simulink model "Eigth_Bit_Adder"  (R2023a)
settings: Solver=VariableStepAuto  StartTime=0.0  StopTime=10.0  RelTol=1e-3
settings Model: Creator=MAN  LastModifiedBy=MAN

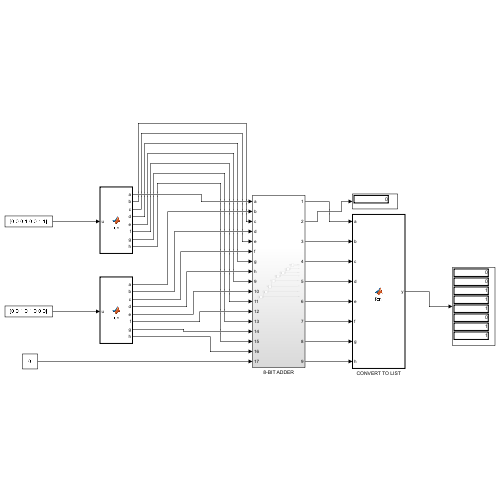
[thumbnail: Simulink's stored preview of the top-level diagram]
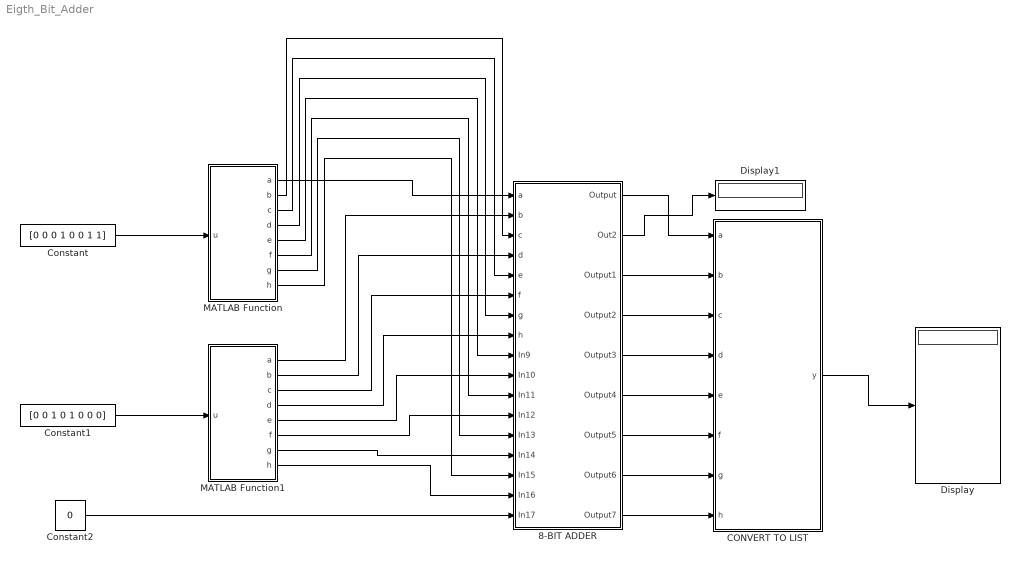
== system Eigth_Bit_Adder ==
  8-BIT ADDER : Subsystem
  CONVERT TO LIST : MATLAB Function  TreatAsAtomicUnit=on
  Constant : Constant  Value=[0 0 0 1 0 0 1 1]
  Constant1 : Constant  Value=[0 0 1 0 1 0 0 0]
  Constant2 : Constant  Value=0
  Display : Display
  Display1 : Display
  MATLAB Function : MATLAB Function  TreatAsAtomicUnit=on
  MATLAB Function1 : MATLAB Function  TreatAsAtomicUnit=on
  wires:
  CONVERT TO LIST/1(y) -> Display/1
  Constant2/1 -> 8-BIT ADDER/17(In17)
  8-BIT ADDER/1(Output) -> CONVERT TO LIST/1(a)
  8-BIT ADDER/3(Output1) -> CONVERT TO LIST/2(b)
  8-BIT ADDER/4(Output2) -> CONVERT TO LIST/3(c)
  8-BIT ADDER/5(Output3) -> CONVERT TO LIST/4(d)
  8-BIT ADDER/6(Output4) -> CONVERT TO LIST/5(e)
  8-BIT ADDER/7(Output5) -> CONVERT TO LIST/6(f)
  8-BIT ADDER/8(Output6) -> CONVERT TO LIST/7(g)
  8-BIT ADDER/9(Output7) -> CONVERT TO LIST/8(h)
  8-BIT ADDER/2(Out2) -> Display1/1
  MATLAB Function/1(a) -> 8-BIT ADDER/1(a)
  MATLAB Function1/1(a) -> 8-BIT ADDER/2(b)
  MATLAB Function/2(b) -> 8-BIT ADDER/3(c)
  MATLAB Function1/2(b) -> 8-BIT ADDER/4(d)
  MATLAB Function/3(c) -> 8-BIT ADDER/5(e)
  MATLAB Function1/3(c) -> 8-BIT ADDER/6(f)
  MATLAB Function/4(d) -> 8-BIT ADDER/7(g)
  MATLAB Function1/4(d) -> 8-BIT ADDER/8(h)
  MATLAB Function/5(e) -> 8-BIT ADDER/9(In9)
  MATLAB Function1/5(e) -> 8-BIT ADDER/10(In10)
  MATLAB Function/6(f) -> 8-BIT ADDER/11(In11)
  MATLAB Function1/6(f) -> 8-BIT ADDER/12(In12)
  MATLAB Function/7(g) -> 8-BIT ADDER/13(In13)
  MATLAB Function1/7(g) -> 8-BIT ADDER/14(In14)
  MATLAB Function/8(h) -> 8-BIT ADDER/15(In15)
  MATLAB Function1/8(h) -> 8-BIT ADDER/16(In16)
  Constant/1 -> MATLAB Function/1(u)
  Constant1/1 -> MATLAB Function1/1(u)

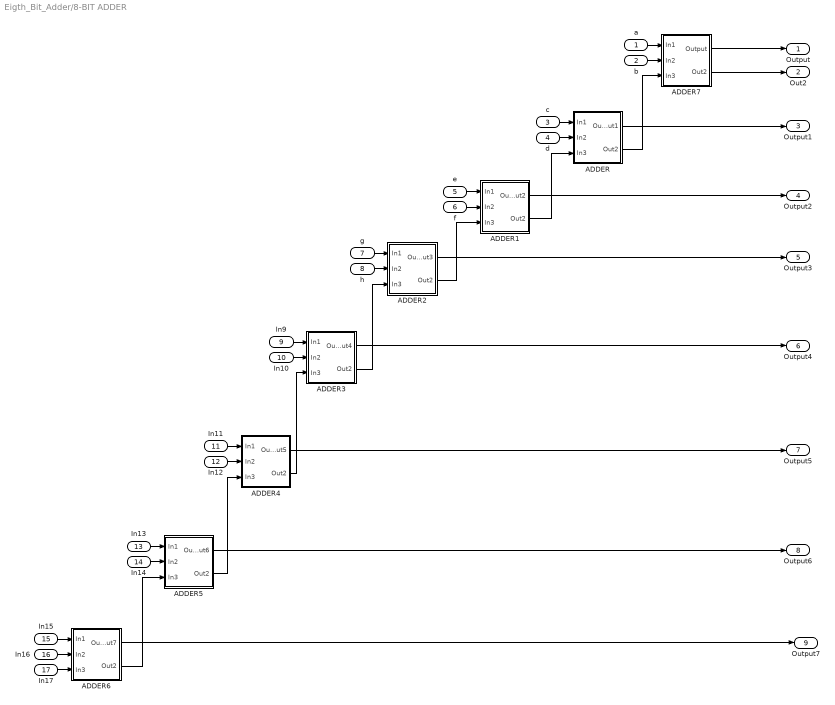
== system Eigth_Bit_Adder/8-BIT ADDER ==
  a : Inport
  b : Inport  Port=2
  c : Inport  Port=3
  d : Inport  Port=4
  e : Inport  Port=5
  f : Inport  Port=6
  g : Inport  Port=7
  h : Inport  Port=8
  In9 : Inport  Port=9
  In10 : Inport  Port=10
  In11 : Inport  Port=11
  In12 : Inport  Port=12
  In13 : Inport  Port=13
  In14 : Inport  Port=14
  In15 : Inport  Port=15
  In16 : Inport  Port=16
  In17 : Inport  Port=17
  ADDER : Subsystem
  ADDER1 : Subsystem
  ADDER2 : Subsystem
  ADDER3 : Subsystem
  ADDER4 : Subsystem
  ADDER5 : Subsystem
  ADDER6 : Subsystem
  ADDER7 : Subsystem
  Output : Outport
  Out2 : Outport  Port=2
  Output1 : Outport  Port=3
  Output2 : Outport  Port=4
  Output3 : Outport  Port=5
  Output4 : Outport  Port=6
  Output5 : Outport  Port=7
  Output6 : Outport  Port=8
  Output7 : Outport  Port=9
  wires:
  ADDER3/1(Output4) -> Output4/1
  ADDER1/2(Out2) -> ADDER/3(In3)
  h/1 -> ADDER2/2(In2)
  In17/1 -> ADDER6/3(In3)
  ADDER/1(Output1) -> Output1/1
  ADDER2/2(Out2) -> ADDER1/3(In3)
  ADDER6/2(Out2) -> ADDER5/3(In3)
  ADDER3/2(Out2) -> ADDER2/3(In3)
  In16/1 -> ADDER6/2(In2)
  ADDER4/2(Out2) -> ADDER3/3(In3)
  In10/1 -> ADDER3/2(In2)
  ADDER5/2(Out2) -> ADDER4/3(In3)
  ADDER2/1(Output3) -> Output3/1
  In14/1 -> ADDER5/2(In2)
  ADDER6/1(Output7) -> Output7/1
  ADDER/2(Out2) -> ADDER7/3(In3)
  ADDER5/1(Output6) -> Output6/1
  ADDER1/1(Output2) -> Output2/1
  f/1 -> ADDER1/2(In2)
  In9/1 -> ADDER3/1(In1)
  e/1 -> ADDER1/1(In1)
  c/1 -> ADDER/1(In1)
  ADDER7/1(Output) -> Output/1
  g/1 -> ADDER2/1(In1)
  d/1 -> ADDER/2(In2)
  a/1 -> ADDER7/1(In1)
  b/1 -> ADDER7/2(In2)
  In12/1 -> ADDER4/2(In2)
  ADDER7/2(Out2) -> Out2/1
  In15/1 -> ADDER6/1(In1)
  In11/1 -> ADDER4/1(In1)
  In13/1 -> ADDER5/1(In1)
  ADDER4/1(Output5) -> Output5/1

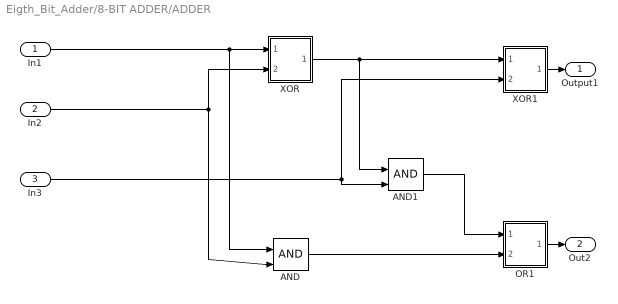
== system Eigth_Bit_Adder/8-BIT ADDER/ADDER ==
  In1 : Inport
  In2 : Inport  Port=2
  In3 : Inport  Port=3
  AND : Logic  IconShape=distinctive  AllPortsSameDT=off  OutDataTypeStr=boolean
  AND1 : Logic  IconShape=distinctive  AllPortsSameDT=off  OutDataTypeStr=boolean
  OR1 : Subsystem
  XOR : Subsystem
  XOR1 : Subsystem
  Output1 : Outport
  Out2 : Outport  Port=2
  wires:
  XOR/1(Out1) -> AND1/1, XOR1/1(In1)
  AND/1 -> OR1/2(In2)
  In2/1 -> XOR/2(In2), AND/2
  In3/1 -> XOR1/2(In2), AND1/2
  In1/1 -> AND/1, XOR/1(In1)
  OR1/1(Out1) -> Out2/1
  AND1/1 -> OR1/1(In1)
  XOR1/1(Out1) -> Output1/1

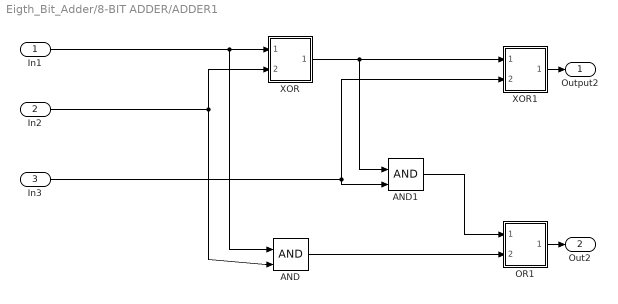
== system Eigth_Bit_Adder/8-BIT ADDER/ADDER1 ==
  In1 : Inport
  In2 : Inport  Port=2
  In3 : Inport  Port=3
  AND : Logic  IconShape=distinctive  AllPortsSameDT=off  OutDataTypeStr=boolean
  AND1 : Logic  IconShape=distinctive  AllPortsSameDT=off  OutDataTypeStr=boolean
  OR1 : Subsystem
  XOR : Subsystem
  XOR1 : Subsystem
  Output2 : Outport
  Out2 : Outport  Port=2
  wires:
  XOR/1(Out1) -> AND1/1, XOR1/1(In1)
  AND/1 -> OR1/2(In2)
  In2/1 -> XOR/2(In2), AND/2
  In3/1 -> XOR1/2(In2), AND1/2
  In1/1 -> AND/1, XOR/1(In1)
  OR1/1(Out1) -> Out2/1
  AND1/1 -> OR1/1(In1)
  XOR1/1(Out1) -> Output2/1

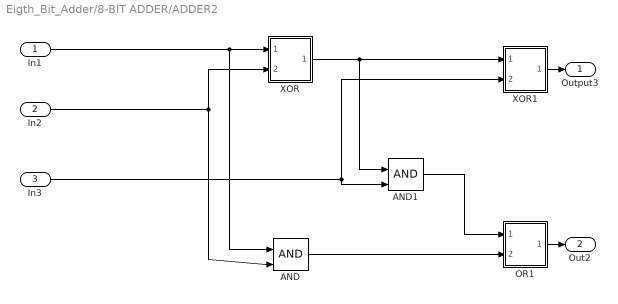
== system Eigth_Bit_Adder/8-BIT ADDER/ADDER2 ==
  In1 : Inport
  In2 : Inport  Port=2
  In3 : Inport  Port=3
  AND : Logic  IconShape=distinctive  AllPortsSameDT=off  OutDataTypeStr=boolean
  AND1 : Logic  IconShape=distinctive  AllPortsSameDT=off  OutDataTypeStr=boolean
  OR1 : Subsystem
  XOR : Subsystem
  XOR1 : Subsystem
  Output3 : Outport
  Out2 : Outport  Port=2
  wires:
  XOR/1(Out1) -> AND1/1, XOR1/1(In1)
  AND/1 -> OR1/2(In2)
  In2/1 -> XOR/2(In2), AND/2
  In3/1 -> XOR1/2(In2), AND1/2
  In1/1 -> AND/1, XOR/1(In1)
  OR1/1(Out1) -> Out2/1
  AND1/1 -> OR1/1(In1)
  XOR1/1(Out1) -> Output3/1

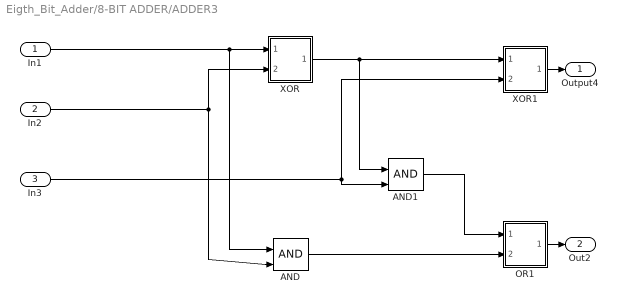
== system Eigth_Bit_Adder/8-BIT ADDER/ADDER3 ==
  In1 : Inport
  In2 : Inport  Port=2
  In3 : Inport  Port=3
  AND : Logic  IconShape=distinctive  AllPortsSameDT=off  OutDataTypeStr=boolean
  AND1 : Logic  IconShape=distinctive  AllPortsSameDT=off  OutDataTypeStr=boolean
  OR1 : Subsystem
  XOR : Subsystem
  XOR1 : Subsystem
  Output4 : Outport
  Out2 : Outport  Port=2
  wires:
  XOR/1(Out1) -> AND1/1, XOR1/1(In1)
  AND/1 -> OR1/2(In2)
  In2/1 -> XOR/2(In2), AND/2
  In3/1 -> XOR1/2(In2), AND1/2
  In1/1 -> AND/1, XOR/1(In1)
  OR1/1(Out1) -> Out2/1
  AND1/1 -> OR1/1(In1)
  XOR1/1(Out1) -> Output4/1

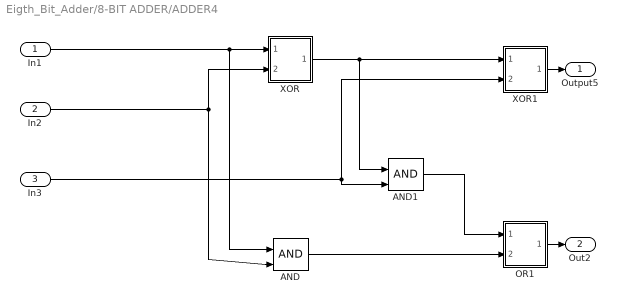
== system Eigth_Bit_Adder/8-BIT ADDER/ADDER4 ==
  In1 : Inport
  In2 : Inport  Port=2
  In3 : Inport  Port=3
  AND : Logic  IconShape=distinctive  AllPortsSameDT=off  OutDataTypeStr=boolean
  AND1 : Logic  IconShape=distinctive  AllPortsSameDT=off  OutDataTypeStr=boolean
  OR1 : Subsystem
  XOR : Subsystem
  XOR1 : Subsystem
  Output5 : Outport
  Out2 : Outport  Port=2
  wires:
  XOR/1(Out1) -> AND1/1, XOR1/1(In1)
  AND/1 -> OR1/2(In2)
  In2/1 -> XOR/2(In2), AND/2
  In3/1 -> XOR1/2(In2), AND1/2
  In1/1 -> AND/1, XOR/1(In1)
  OR1/1(Out1) -> Out2/1
  AND1/1 -> OR1/1(In1)
  XOR1/1(Out1) -> Output5/1

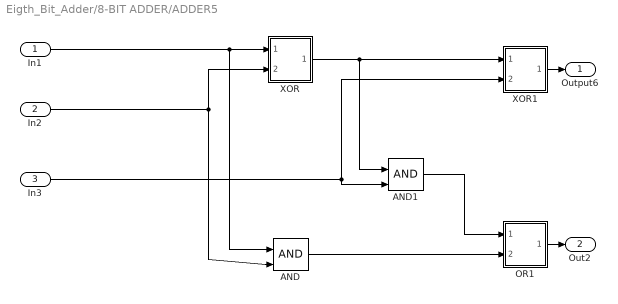
== system Eigth_Bit_Adder/8-BIT ADDER/ADDER5 ==
  In1 : Inport
  In2 : Inport  Port=2
  In3 : Inport  Port=3
  AND : Logic  IconShape=distinctive  AllPortsSameDT=off  OutDataTypeStr=boolean
  AND1 : Logic  IconShape=distinctive  AllPortsSameDT=off  OutDataTypeStr=boolean
  OR1 : Subsystem
  XOR : Subsystem
  XOR1 : Subsystem
  Output6 : Outport
  Out2 : Outport  Port=2
  wires:
  XOR/1(Out1) -> AND1/1, XOR1/1(In1)
  AND/1 -> OR1/2(In2)
  In2/1 -> XOR/2(In2), AND/2
  In3/1 -> XOR1/2(In2), AND1/2
  In1/1 -> AND/1, XOR/1(In1)
  OR1/1(Out1) -> Out2/1
  AND1/1 -> OR1/1(In1)
  XOR1/1(Out1) -> Output6/1

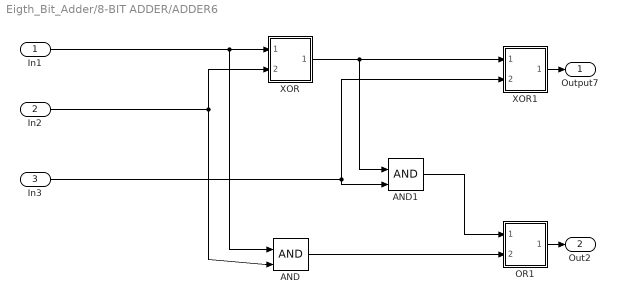
== system Eigth_Bit_Adder/8-BIT ADDER/ADDER6 ==
  In1 : Inport
  In2 : Inport  Port=2
  In3 : Inport  Port=3
  AND : Logic  IconShape=distinctive  AllPortsSameDT=off  OutDataTypeStr=boolean
  AND1 : Logic  IconShape=distinctive  AllPortsSameDT=off  OutDataTypeStr=boolean
  OR1 : Subsystem
  XOR : Subsystem
  XOR1 : Subsystem
  Output7 : Outport
  Out2 : Outport  Port=2
  wires:
  XOR/1(Out1) -> AND1/1, XOR1/1(In1)
  AND/1 -> OR1/2(In2)
  In2/1 -> XOR/2(In2), AND/2
  In3/1 -> XOR1/2(In2), AND1/2
  In1/1 -> AND/1, XOR/1(In1)
  OR1/1(Out1) -> Out2/1
  AND1/1 -> OR1/1(In1)
  XOR1/1(Out1) -> Output7/1

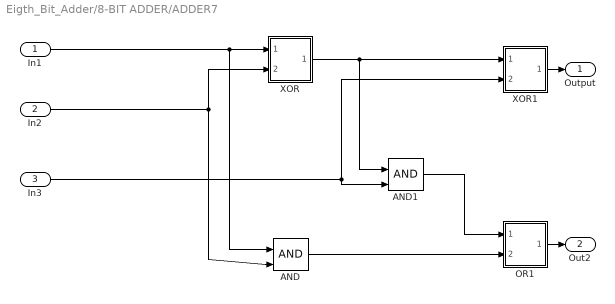
== system Eigth_Bit_Adder/8-BIT ADDER/ADDER7 ==
  In1 : Inport
  In2 : Inport  Port=2
  In3 : Inport  Port=3
  AND : Logic  IconShape=distinctive  AllPortsSameDT=off  OutDataTypeStr=boolean
  AND1 : Logic  IconShape=distinctive  AllPortsSameDT=off  OutDataTypeStr=boolean
  OR1 : Subsystem
  XOR : Subsystem
  XOR1 : Subsystem
  Output : Outport
  Out2 : Outport  Port=2
  wires:
  XOR/1(Out1) -> AND1/1, XOR1/1(In1)
  AND/1 -> OR1/2(In2)
  In2/1 -> XOR/2(In2), AND/2
  In3/1 -> XOR1/2(In2), AND1/2
  In1/1 -> AND/1, XOR/1(In1)
  OR1/1(Out1) -> Out2/1
  AND1/1 -> OR1/1(In1)
  XOR1/1(Out1) -> Output/1

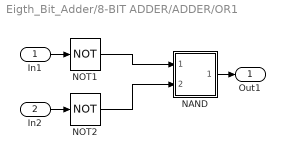
== system Eigth_Bit_Adder/8-BIT ADDER/ADDER/OR1 ==
  In1 : Inport
  In2 : Inport  Port=2
  NAND : Subsystem
  NOT1 : Logic  Operator=NOT  IconShape=distinctive  AllPortsSameDT=off  OutDataTypeStr=boolean
  NOT2 : Logic  Operator=NOT  IconShape=distinctive  AllPortsSameDT=off  OutDataTypeStr=boolean
  Out1 : Outport
  wires:
  In1/1 -> NOT1/1
  In2/1 -> NOT2/1
  NOT1/1 -> NAND/1(In1)
  NOT2/1 -> NAND/2(In2)
  NAND/1(Out1) -> Out1/1

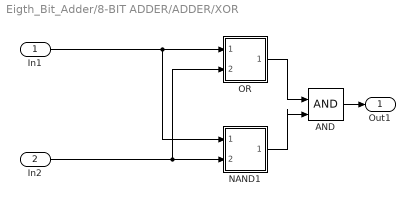
== system Eigth_Bit_Adder/8-BIT ADDER/ADDER/XOR ==
  In1 : Inport
  In2 : Inport  Port=2
  AND : Logic  IconShape=distinctive  AllPortsSameDT=off  OutDataTypeStr=boolean
  NAND1 : Subsystem
  OR : Subsystem
  Out1 : Outport
  wires:
  In2/1 -> NAND1/2(In2), OR/2(In2)
  In1/1 -> NAND1/1(In1), OR/1(In1)
  NAND1/1(Out1) -> AND/2
  AND/1 -> Out1/1
  OR/1(Out1) -> AND/1

== system Eigth_Bit_Adder/8-BIT ADDER/ADDER/XOR1 ==
  In1 : Inport
  In2 : Inport  Port=2
  AND : Logic  IconShape=distinctive  AllPortsSameDT=off  OutDataTypeStr=boolean
  NAND1 : Subsystem
  OR : Subsystem
  Out1 : Outport
  wires:
  In2/1 -> NAND1/2(In2), OR/2(In2)
  In1/1 -> NAND1/1(In1), OR/1(In1)
  NAND1/1(Out1) -> AND/2
  AND/1 -> Out1/1
  OR/1(Out1) -> AND/1

== system Eigth_Bit_Adder/8-BIT ADDER/ADDER1/OR1 ==
  In1 : Inport
  In2 : Inport  Port=2
  NAND : Subsystem
  NOT1 : Logic  Operator=NOT  IconShape=distinctive  AllPortsSameDT=off  OutDataTypeStr=boolean
  NOT2 : Logic  Operator=NOT  IconShape=distinctive  AllPortsSameDT=off  OutDataTypeStr=boolean
  Out1 : Outport
  wires:
  In1/1 -> NOT1/1
  In2/1 -> NOT2/1
  NOT1/1 -> NAND/1(In1)
  NOT2/1 -> NAND/2(In2)
  NAND/1(Out1) -> Out1/1

== system Eigth_Bit_Adder/8-BIT ADDER/ADDER1/XOR ==
  In1 : Inport
  In2 : Inport  Port=2
  AND : Logic  IconShape=distinctive  AllPortsSameDT=off  OutDataTypeStr=boolean
  NAND1 : Subsystem
  OR : Subsystem
  Out1 : Outport
  wires:
  In2/1 -> NAND1/2(In2), OR/2(In2)
  In1/1 -> NAND1/1(In1), OR/1(In1)
  NAND1/1(Out1) -> AND/2
  AND/1 -> Out1/1
  OR/1(Out1) -> AND/1

== system Eigth_Bit_Adder/8-BIT ADDER/ADDER1/XOR1 ==
  In1 : Inport
  In2 : Inport  Port=2
  AND : Logic  IconShape=distinctive  AllPortsSameDT=off  OutDataTypeStr=boolean
  NAND1 : Subsystem
  OR : Subsystem
  Out1 : Outport
  wires:
  In2/1 -> NAND1/2(In2), OR/2(In2)
  In1/1 -> NAND1/1(In1), OR/1(In1)
  NAND1/1(Out1) -> AND/2
  AND/1 -> Out1/1
  OR/1(Out1) -> AND/1

== system Eigth_Bit_Adder/8-BIT ADDER/ADDER2/OR1 ==
  In1 : Inport
  In2 : Inport  Port=2
  NAND : Subsystem
  NOT1 : Logic  Operator=NOT  IconShape=distinctive  AllPortsSameDT=off  OutDataTypeStr=boolean
  NOT2 : Logic  Operator=NOT  IconShape=distinctive  AllPortsSameDT=off  OutDataTypeStr=boolean
  Out1 : Outport
  wires:
  In1/1 -> NOT1/1
  In2/1 -> NOT2/1
  NOT1/1 -> NAND/1(In1)
  NOT2/1 -> NAND/2(In2)
  NAND/1(Out1) -> Out1/1

== system Eigth_Bit_Adder/8-BIT ADDER/ADDER2/XOR ==
  In1 : Inport
  In2 : Inport  Port=2
  AND : Logic  IconShape=distinctive  AllPortsSameDT=off  OutDataTypeStr=boolean
  NAND1 : Subsystem
  OR : Subsystem
  Out1 : Outport
  wires:
  In2/1 -> NAND1/2(In2), OR/2(In2)
  In1/1 -> NAND1/1(In1), OR/1(In1)
  NAND1/1(Out1) -> AND/2
  AND/1 -> Out1/1
  OR/1(Out1) -> AND/1

== system Eigth_Bit_Adder/8-BIT ADDER/ADDER2/XOR1 ==
  In1 : Inport
  In2 : Inport  Port=2
  AND : Logic  IconShape=distinctive  AllPortsSameDT=off  OutDataTypeStr=boolean
  NAND1 : Subsystem
  OR : Subsystem
  Out1 : Outport
  wires:
  In2/1 -> NAND1/2(In2), OR/2(In2)
  In1/1 -> NAND1/1(In1), OR/1(In1)
  NAND1/1(Out1) -> AND/2
  AND/1 -> Out1/1
  OR/1(Out1) -> AND/1

== system Eigth_Bit_Adder/8-BIT ADDER/ADDER3/OR1 ==
  In1 : Inport
  In2 : Inport  Port=2
  NAND : Subsystem
  NOT1 : Logic  Operator=NOT  IconShape=distinctive  AllPortsSameDT=off  OutDataTypeStr=boolean
  NOT2 : Logic  Operator=NOT  IconShape=distinctive  AllPortsSameDT=off  OutDataTypeStr=boolean
  Out1 : Outport
  wires:
  In1/1 -> NOT1/1
  In2/1 -> NOT2/1
  NOT1/1 -> NAND/1(In1)
  NOT2/1 -> NAND/2(In2)
  NAND/1(Out1) -> Out1/1

== system Eigth_Bit_Adder/8-BIT ADDER/ADDER3/XOR ==
  In1 : Inport
  In2 : Inport  Port=2
  AND : Logic  IconShape=distinctive  AllPortsSameDT=off  OutDataTypeStr=boolean
  NAND1 : Subsystem
  OR : Subsystem
  Out1 : Outport
  wires:
  In2/1 -> NAND1/2(In2), OR/2(In2)
  In1/1 -> NAND1/1(In1), OR/1(In1)
  NAND1/1(Out1) -> AND/2
  AND/1 -> Out1/1
  OR/1(Out1) -> AND/1

== system Eigth_Bit_Adder/8-BIT ADDER/ADDER3/XOR1 ==
  In1 : Inport
  In2 : Inport  Port=2
  AND : Logic  IconShape=distinctive  AllPortsSameDT=off  OutDataTypeStr=boolean
  NAND1 : Subsystem
  OR : Subsystem
  Out1 : Outport
  wires:
  In2/1 -> NAND1/2(In2), OR/2(In2)
  In1/1 -> NAND1/1(In1), OR/1(In1)
  NAND1/1(Out1) -> AND/2
  AND/1 -> Out1/1
  OR/1(Out1) -> AND/1

== system Eigth_Bit_Adder/8-BIT ADDER/ADDER4/OR1 ==
  In1 : Inport
  In2 : Inport  Port=2
  NAND : Subsystem
  NOT1 : Logic  Operator=NOT  IconShape=distinctive  AllPortsSameDT=off  OutDataTypeStr=boolean
  NOT2 : Logic  Operator=NOT  IconShape=distinctive  AllPortsSameDT=off  OutDataTypeStr=boolean
  Out1 : Outport
  wires:
  In1/1 -> NOT1/1
  In2/1 -> NOT2/1
  NOT1/1 -> NAND/1(In1)
  NOT2/1 -> NAND/2(In2)
  NAND/1(Out1) -> Out1/1

== system Eigth_Bit_Adder/8-BIT ADDER/ADDER4/XOR ==
  In1 : Inport
  In2 : Inport  Port=2
  AND : Logic  IconShape=distinctive  AllPortsSameDT=off  OutDataTypeStr=boolean
  NAND1 : Subsystem
  OR : Subsystem
  Out1 : Outport
  wires:
  In2/1 -> NAND1/2(In2), OR/2(In2)
  In1/1 -> NAND1/1(In1), OR/1(In1)
  NAND1/1(Out1) -> AND/2
  AND/1 -> Out1/1
  OR/1(Out1) -> AND/1

== system Eigth_Bit_Adder/8-BIT ADDER/ADDER4/XOR1 ==
  In1 : Inport
  In2 : Inport  Port=2
  AND : Logic  IconShape=distinctive  AllPortsSameDT=off  OutDataTypeStr=boolean
  NAND1 : Subsystem
  OR : Subsystem
  Out1 : Outport
  wires:
  In2/1 -> NAND1/2(In2), OR/2(In2)
  In1/1 -> NAND1/1(In1), OR/1(In1)
  NAND1/1(Out1) -> AND/2
  AND/1 -> Out1/1
  OR/1(Out1) -> AND/1

== system Eigth_Bit_Adder/8-BIT ADDER/ADDER5/OR1 ==
  In1 : Inport
  In2 : Inport  Port=2
  NAND : Subsystem
  NOT1 : Logic  Operator=NOT  IconShape=distinctive  AllPortsSameDT=off  OutDataTypeStr=boolean
  NOT2 : Logic  Operator=NOT  IconShape=distinctive  AllPortsSameDT=off  OutDataTypeStr=boolean
  Out1 : Outport
  wires:
  In1/1 -> NOT1/1
  In2/1 -> NOT2/1
  NOT1/1 -> NAND/1(In1)
  NOT2/1 -> NAND/2(In2)
  NAND/1(Out1) -> Out1/1

== system Eigth_Bit_Adder/8-BIT ADDER/ADDER5/XOR ==
  In1 : Inport
  In2 : Inport  Port=2
  AND : Logic  IconShape=distinctive  AllPortsSameDT=off  OutDataTypeStr=boolean
  NAND1 : Subsystem
  OR : Subsystem
  Out1 : Outport
  wires:
  In2/1 -> NAND1/2(In2), OR/2(In2)
  In1/1 -> NAND1/1(In1), OR/1(In1)
  NAND1/1(Out1) -> AND/2
  AND/1 -> Out1/1
  OR/1(Out1) -> AND/1

== system Eigth_Bit_Adder/8-BIT ADDER/ADDER5/XOR1 ==
  In1 : Inport
  In2 : Inport  Port=2
  AND : Logic  IconShape=distinctive  AllPortsSameDT=off  OutDataTypeStr=boolean
  NAND1 : Subsystem
  OR : Subsystem
  Out1 : Outport
  wires:
  In2/1 -> NAND1/2(In2), OR/2(In2)
  In1/1 -> NAND1/1(In1), OR/1(In1)
  NAND1/1(Out1) -> AND/2
  AND/1 -> Out1/1
  OR/1(Out1) -> AND/1

== system Eigth_Bit_Adder/8-BIT ADDER/ADDER6/OR1 ==
  In1 : Inport
  In2 : Inport  Port=2
  NAND : Subsystem
  NOT1 : Logic  Operator=NOT  IconShape=distinctive  AllPortsSameDT=off  OutDataTypeStr=boolean
  NOT2 : Logic  Operator=NOT  IconShape=distinctive  AllPortsSameDT=off  OutDataTypeStr=boolean
  Out1 : Outport
  wires:
  In1/1 -> NOT1/1
  In2/1 -> NOT2/1
  NOT1/1 -> NAND/1(In1)
  NOT2/1 -> NAND/2(In2)
  NAND/1(Out1) -> Out1/1

== system Eigth_Bit_Adder/8-BIT ADDER/ADDER6/XOR ==
  In1 : Inport
  In2 : Inport  Port=2
  AND : Logic  IconShape=distinctive  AllPortsSameDT=off  OutDataTypeStr=boolean
  NAND1 : Subsystem
  OR : Subsystem
  Out1 : Outport
  wires:
  In2/1 -> NAND1/2(In2), OR/2(In2)
  In1/1 -> NAND1/1(In1), OR/1(In1)
  NAND1/1(Out1) -> AND/2
  AND/1 -> Out1/1
  OR/1(Out1) -> AND/1

== system Eigth_Bit_Adder/8-BIT ADDER/ADDER6/XOR1 ==
  In1 : Inport
  In2 : Inport  Port=2
  AND : Logic  IconShape=distinctive  AllPortsSameDT=off  OutDataTypeStr=boolean
  NAND1 : Subsystem
  OR : Subsystem
  Out1 : Outport
  wires:
  In2/1 -> NAND1/2(In2), OR/2(In2)
  In1/1 -> NAND1/1(In1), OR/1(In1)
  NAND1/1(Out1) -> AND/2
  AND/1 -> Out1/1
  OR/1(Out1) -> AND/1

== system Eigth_Bit_Adder/8-BIT ADDER/ADDER7/OR1 ==
  In1 : Inport
  In2 : Inport  Port=2
  NAND : Subsystem
  NOT1 : Logic  Operator=NOT  IconShape=distinctive  AllPortsSameDT=off  OutDataTypeStr=boolean
  NOT2 : Logic  Operator=NOT  IconShape=distinctive  AllPortsSameDT=off  OutDataTypeStr=boolean
  Out1 : Outport
  wires:
  In1/1 -> NOT1/1
  In2/1 -> NOT2/1
  NOT1/1 -> NAND/1(In1)
  NOT2/1 -> NAND/2(In2)
  NAND/1(Out1) -> Out1/1

== system Eigth_Bit_Adder/8-BIT ADDER/ADDER7/XOR ==
  In1 : Inport
  In2 : Inport  Port=2
  AND : Logic  IconShape=distinctive  AllPortsSameDT=off  OutDataTypeStr=boolean
  NAND1 : Subsystem
  OR : Subsystem
  Out1 : Outport
  wires:
  In2/1 -> NAND1/2(In2), OR/2(In2)
  In1/1 -> NAND1/1(In1), OR/1(In1)
  NAND1/1(Out1) -> AND/2
  AND/1 -> Out1/1
  OR/1(Out1) -> AND/1

== system Eigth_Bit_Adder/8-BIT ADDER/ADDER7/XOR1 ==
  In1 : Inport
  In2 : Inport  Port=2
  AND : Logic  IconShape=distinctive  AllPortsSameDT=off  OutDataTypeStr=boolean
  NAND1 : Subsystem
  OR : Subsystem
  Out1 : Outport
  wires:
  In2/1 -> NAND1/2(In2), OR/2(In2)
  In1/1 -> NAND1/1(In1), OR/1(In1)
  NAND1/1(Out1) -> AND/2
  AND/1 -> Out1/1
  OR/1(Out1) -> AND/1

== system Eigth_Bit_Adder/8-BIT ADDER/ADDER/OR1/NAND ==
  In1 : Inport
  In2 : Inport  Port=2
  AND : Logic  IconShape=distinctive  AllPortsSameDT=off  OutDataTypeStr=boolean
  NOT : Logic  Operator=NOT  IconShape=distinctive  AllPortsSameDT=off  OutDataTypeStr=boolean
  Out1 : Outport
  wires:
  AND/1 -> NOT/1
  In1/1 -> AND/1
  NOT/1 -> Out1/1
  In2/1 -> AND/2

== system Eigth_Bit_Adder/8-BIT ADDER/ADDER/XOR/NAND1 ==
  In1 : Inport
  In2 : Inport  Port=2
  AND : Logic  IconShape=distinctive  AllPortsSameDT=off  OutDataTypeStr=boolean
  NOT : Logic  Operator=NOT  IconShape=distinctive  AllPortsSameDT=off  OutDataTypeStr=boolean
  Out1 : Outport
  wires:
  In2/1 -> AND/2
  NOT/1 -> Out1/1
  In1/1 -> AND/1
  AND/1 -> NOT/1

== system Eigth_Bit_Adder/8-BIT ADDER/ADDER/XOR/OR ==
  In1 : Inport
  In2 : Inport  Port=2
  NAND : Subsystem
  NOT1 : Logic  Operator=NOT  IconShape=distinctive  AllPortsSameDT=off  OutDataTypeStr=boolean
  NOT2 : Logic  Operator=NOT  IconShape=distinctive  AllPortsSameDT=off  OutDataTypeStr=boolean
  Out1 : Outport
  wires:
  In1/1 -> NOT1/1
  In2/1 -> NOT2/1
  NOT1/1 -> NAND/1(In1)
  NOT2/1 -> NAND/2(In2)
  NAND/1(Out1) -> Out1/1

== system Eigth_Bit_Adder/8-BIT ADDER/ADDER/XOR1/NAND1 ==
  In1 : Inport
  In2 : Inport  Port=2
  AND : Logic  IconShape=distinctive  AllPortsSameDT=off  OutDataTypeStr=boolean
  NOT : Logic  Operator=NOT  IconShape=distinctive  AllPortsSameDT=off  OutDataTypeStr=boolean
  Out1 : Outport
  wires:
  In2/1 -> AND/2
  NOT/1 -> Out1/1
  In1/1 -> AND/1
  AND/1 -> NOT/1

== system Eigth_Bit_Adder/8-BIT ADDER/ADDER/XOR1/OR ==
  In1 : Inport
  In2 : Inport  Port=2
  NAND : Subsystem
  NOT1 : Logic  Operator=NOT  IconShape=distinctive  AllPortsSameDT=off  OutDataTypeStr=boolean
  NOT2 : Logic  Operator=NOT  IconShape=distinctive  AllPortsSameDT=off  OutDataTypeStr=boolean
  Out1 : Outport
  wires:
  In1/1 -> NOT1/1
  In2/1 -> NOT2/1
  NOT1/1 -> NAND/1(In1)
  NOT2/1 -> NAND/2(In2)
  NAND/1(Out1) -> Out1/1

== system Eigth_Bit_Adder/8-BIT ADDER/ADDER1/OR1/NAND ==
  In1 : Inport
  In2 : Inport  Port=2
  AND : Logic  IconShape=distinctive  AllPortsSameDT=off  OutDataTypeStr=boolean
  NOT : Logic  Operator=NOT  IconShape=distinctive  AllPortsSameDT=off  OutDataTypeStr=boolean
  Out1 : Outport
  wires:
  AND/1 -> NOT/1
  In1/1 -> AND/1
  NOT/1 -> Out1/1
  In2/1 -> AND/2

== system Eigth_Bit_Adder/8-BIT ADDER/ADDER1/XOR/NAND1 ==
  In1 : Inport
  In2 : Inport  Port=2
  AND : Logic  IconShape=distinctive  AllPortsSameDT=off  OutDataTypeStr=boolean
  NOT : Logic  Operator=NOT  IconShape=distinctive  AllPortsSameDT=off  OutDataTypeStr=boolean
  Out1 : Outport
  wires:
  In2/1 -> AND/2
  NOT/1 -> Out1/1
  In1/1 -> AND/1
  AND/1 -> NOT/1

== system Eigth_Bit_Adder/8-BIT ADDER/ADDER1/XOR/OR ==
  In1 : Inport
  In2 : Inport  Port=2
  NAND : Subsystem
  NOT1 : Logic  Operator=NOT  IconShape=distinctive  AllPortsSameDT=off  OutDataTypeStr=boolean
  NOT2 : Logic  Operator=NOT  IconShape=distinctive  AllPortsSameDT=off  OutDataTypeStr=boolean
  Out1 : Outport
  wires:
  In1/1 -> NOT1/1
  In2/1 -> NOT2/1
  NOT1/1 -> NAND/1(In1)
  NOT2/1 -> NAND/2(In2)
  NAND/1(Out1) -> Out1/1

== system Eigth_Bit_Adder/8-BIT ADDER/ADDER1/XOR1/NAND1 ==
  In1 : Inport
  In2 : Inport  Port=2
  AND : Logic  IconShape=distinctive  AllPortsSameDT=off  OutDataTypeStr=boolean
  NOT : Logic  Operator=NOT  IconShape=distinctive  AllPortsSameDT=off  OutDataTypeStr=boolean
  Out1 : Outport
  wires:
  In2/1 -> AND/2
  NOT/1 -> Out1/1
  In1/1 -> AND/1
  AND/1 -> NOT/1

== system Eigth_Bit_Adder/8-BIT ADDER/ADDER1/XOR1/OR ==
  In1 : Inport
  In2 : Inport  Port=2
  NAND : Subsystem
  NOT1 : Logic  Operator=NOT  IconShape=distinctive  AllPortsSameDT=off  OutDataTypeStr=boolean
  NOT2 : Logic  Operator=NOT  IconShape=distinctive  AllPortsSameDT=off  OutDataTypeStr=boolean
  Out1 : Outport
  wires:
  In1/1 -> NOT1/1
  In2/1 -> NOT2/1
  NOT1/1 -> NAND/1(In1)
  NOT2/1 -> NAND/2(In2)
  NAND/1(Out1) -> Out1/1

== system Eigth_Bit_Adder/8-BIT ADDER/ADDER2/OR1/NAND ==
  In1 : Inport
  In2 : Inport  Port=2
  AND : Logic  IconShape=distinctive  AllPortsSameDT=off  OutDataTypeStr=boolean
  NOT : Logic  Operator=NOT  IconShape=distinctive  AllPortsSameDT=off  OutDataTypeStr=boolean
  Out1 : Outport
  wires:
  AND/1 -> NOT/1
  In1/1 -> AND/1
  NOT/1 -> Out1/1
  In2/1 -> AND/2

== system Eigth_Bit_Adder/8-BIT ADDER/ADDER2/XOR/NAND1 ==
  In1 : Inport
  In2 : Inport  Port=2
  AND : Logic  IconShape=distinctive  AllPortsSameDT=off  OutDataTypeStr=boolean
  NOT : Logic  Operator=NOT  IconShape=distinctive  AllPortsSameDT=off  OutDataTypeStr=boolean
  Out1 : Outport
  wires:
  In2/1 -> AND/2
  NOT/1 -> Out1/1
  In1/1 -> AND/1
  AND/1 -> NOT/1

== system Eigth_Bit_Adder/8-BIT ADDER/ADDER2/XOR/OR ==
  In1 : Inport
  In2 : Inport  Port=2
  NAND : Subsystem
  NOT1 : Logic  Operator=NOT  IconShape=distinctive  AllPortsSameDT=off  OutDataTypeStr=boolean
  NOT2 : Logic  Operator=NOT  IconShape=distinctive  AllPortsSameDT=off  OutDataTypeStr=boolean
  Out1 : Outport
  wires:
  In1/1 -> NOT1/1
  In2/1 -> NOT2/1
  NOT1/1 -> NAND/1(In1)
  NOT2/1 -> NAND/2(In2)
  NAND/1(Out1) -> Out1/1

== system Eigth_Bit_Adder/8-BIT ADDER/ADDER2/XOR1/NAND1 ==
  In1 : Inport
  In2 : Inport  Port=2
  AND : Logic  IconShape=distinctive  AllPortsSameDT=off  OutDataTypeStr=boolean
  NOT : Logic  Operator=NOT  IconShape=distinctive  AllPortsSameDT=off  OutDataTypeStr=boolean
  Out1 : Outport
  wires:
  In2/1 -> AND/2
  NOT/1 -> Out1/1
  In1/1 -> AND/1
  AND/1 -> NOT/1

== system Eigth_Bit_Adder/8-BIT ADDER/ADDER2/XOR1/OR ==
  In1 : Inport
  In2 : Inport  Port=2
  NAND : Subsystem
  NOT1 : Logic  Operator=NOT  IconShape=distinctive  AllPortsSameDT=off  OutDataTypeStr=boolean
  NOT2 : Logic  Operator=NOT  IconShape=distinctive  AllPortsSameDT=off  OutDataTypeStr=boolean
  Out1 : Outport
  wires:
  In1/1 -> NOT1/1
  In2/1 -> NOT2/1
  NOT1/1 -> NAND/1(In1)
  NOT2/1 -> NAND/2(In2)
  NAND/1(Out1) -> Out1/1

== system Eigth_Bit_Adder/8-BIT ADDER/ADDER3/OR1/NAND ==
  In1 : Inport
  In2 : Inport  Port=2
  AND : Logic  IconShape=distinctive  AllPortsSameDT=off  OutDataTypeStr=boolean
  NOT : Logic  Operator=NOT  IconShape=distinctive  AllPortsSameDT=off  OutDataTypeStr=boolean
  Out1 : Outport
  wires:
  AND/1 -> NOT/1
  In1/1 -> AND/1
  NOT/1 -> Out1/1
  In2/1 -> AND/2

== system Eigth_Bit_Adder/8-BIT ADDER/ADDER3/XOR/NAND1 ==
  In1 : Inport
  In2 : Inport  Port=2
  AND : Logic  IconShape=distinctive  AllPortsSameDT=off  OutDataTypeStr=boolean
  NOT : Logic  Operator=NOT  IconShape=distinctive  AllPortsSameDT=off  OutDataTypeStr=boolean
  Out1 : Outport
  wires:
  In2/1 -> AND/2
  NOT/1 -> Out1/1
  In1/1 -> AND/1
  AND/1 -> NOT/1

== system Eigth_Bit_Adder/8-BIT ADDER/ADDER3/XOR/OR ==
  In1 : Inport
  In2 : Inport  Port=2
  NAND : Subsystem
  NOT1 : Logic  Operator=NOT  IconShape=distinctive  AllPortsSameDT=off  OutDataTypeStr=boolean
  NOT2 : Logic  Operator=NOT  IconShape=distinctive  AllPortsSameDT=off  OutDataTypeStr=boolean
  Out1 : Outport
  wires:
  In1/1 -> NOT1/1
  In2/1 -> NOT2/1
  NOT1/1 -> NAND/1(In1)
  NOT2/1 -> NAND/2(In2)
  NAND/1(Out1) -> Out1/1

== system Eigth_Bit_Adder/8-BIT ADDER/ADDER3/XOR1/NAND1 ==
  In1 : Inport
  In2 : Inport  Port=2
  AND : Logic  IconShape=distinctive  AllPortsSameDT=off  OutDataTypeStr=boolean
  NOT : Logic  Operator=NOT  IconShape=distinctive  AllPortsSameDT=off  OutDataTypeStr=boolean
  Out1 : Outport
  wires:
  In2/1 -> AND/2
  NOT/1 -> Out1/1
  In1/1 -> AND/1
  AND/1 -> NOT/1

== system Eigth_Bit_Adder/8-BIT ADDER/ADDER3/XOR1/OR ==
  In1 : Inport
  In2 : Inport  Port=2
  NAND : Subsystem
  NOT1 : Logic  Operator=NOT  IconShape=distinctive  AllPortsSameDT=off  OutDataTypeStr=boolean
  NOT2 : Logic  Operator=NOT  IconShape=distinctive  AllPortsSameDT=off  OutDataTypeStr=boolean
  Out1 : Outport
  wires:
  In1/1 -> NOT1/1
  In2/1 -> NOT2/1
  NOT1/1 -> NAND/1(In1)
  NOT2/1 -> NAND/2(In2)
  NAND/1(Out1) -> Out1/1

== system Eigth_Bit_Adder/8-BIT ADDER/ADDER4/OR1/NAND ==
  In1 : Inport
  In2 : Inport  Port=2
  AND : Logic  IconShape=distinctive  AllPortsSameDT=off  OutDataTypeStr=boolean
  NOT : Logic  Operator=NOT  IconShape=distinctive  AllPortsSameDT=off  OutDataTypeStr=boolean
  Out1 : Outport
  wires:
  AND/1 -> NOT/1
  In1/1 -> AND/1
  NOT/1 -> Out1/1
  In2/1 -> AND/2

== system Eigth_Bit_Adder/8-BIT ADDER/ADDER4/XOR/NAND1 ==
  In1 : Inport
  In2 : Inport  Port=2
  AND : Logic  IconShape=distinctive  AllPortsSameDT=off  OutDataTypeStr=boolean
  NOT : Logic  Operator=NOT  IconShape=distinctive  AllPortsSameDT=off  OutDataTypeStr=boolean
  Out1 : Outport
  wires:
  In2/1 -> AND/2
  NOT/1 -> Out1/1
  In1/1 -> AND/1
  AND/1 -> NOT/1

== system Eigth_Bit_Adder/8-BIT ADDER/ADDER4/XOR/OR ==
  In1 : Inport
  In2 : Inport  Port=2
  NAND : Subsystem
  NOT1 : Logic  Operator=NOT  IconShape=distinctive  AllPortsSameDT=off  OutDataTypeStr=boolean
  NOT2 : Logic  Operator=NOT  IconShape=distinctive  AllPortsSameDT=off  OutDataTypeStr=boolean
  Out1 : Outport
  wires:
  In1/1 -> NOT1/1
  In2/1 -> NOT2/1
  NOT1/1 -> NAND/1(In1)
  NOT2/1 -> NAND/2(In2)
  NAND/1(Out1) -> Out1/1

== system Eigth_Bit_Adder/8-BIT ADDER/ADDER4/XOR1/NAND1 ==
  In1 : Inport
  In2 : Inport  Port=2
  AND : Logic  IconShape=distinctive  AllPortsSameDT=off  OutDataTypeStr=boolean
  NOT : Logic  Operator=NOT  IconShape=distinctive  AllPortsSameDT=off  OutDataTypeStr=boolean
  Out1 : Outport
  wires:
  In2/1 -> AND/2
  NOT/1 -> Out1/1
  In1/1 -> AND/1
  AND/1 -> NOT/1

== system Eigth_Bit_Adder/8-BIT ADDER/ADDER4/XOR1/OR ==
  In1 : Inport
  In2 : Inport  Port=2
  NAND : Subsystem
  NOT1 : Logic  Operator=NOT  IconShape=distinctive  AllPortsSameDT=off  OutDataTypeStr=boolean
  NOT2 : Logic  Operator=NOT  IconShape=distinctive  AllPortsSameDT=off  OutDataTypeStr=boolean
  Out1 : Outport
  wires:
  In1/1 -> NOT1/1
  In2/1 -> NOT2/1
  NOT1/1 -> NAND/1(In1)
  NOT2/1 -> NAND/2(In2)
  NAND/1(Out1) -> Out1/1

== system Eigth_Bit_Adder/8-BIT ADDER/ADDER5/OR1/NAND ==
  In1 : Inport
  In2 : Inport  Port=2
  AND : Logic  IconShape=distinctive  AllPortsSameDT=off  OutDataTypeStr=boolean
  NOT : Logic  Operator=NOT  IconShape=distinctive  AllPortsSameDT=off  OutDataTypeStr=boolean
  Out1 : Outport
  wires:
  AND/1 -> NOT/1
  In1/1 -> AND/1
  NOT/1 -> Out1/1
  In2/1 -> AND/2

== system Eigth_Bit_Adder/8-BIT ADDER/ADDER5/XOR/NAND1 ==
  In1 : Inport
  In2 : Inport  Port=2
  AND : Logic  IconShape=distinctive  AllPortsSameDT=off  OutDataTypeStr=boolean
  NOT : Logic  Operator=NOT  IconShape=distinctive  AllPortsSameDT=off  OutDataTypeStr=boolean
  Out1 : Outport
  wires:
  In2/1 -> AND/2
  NOT/1 -> Out1/1
  In1/1 -> AND/1
  AND/1 -> NOT/1

== system Eigth_Bit_Adder/8-BIT ADDER/ADDER5/XOR/OR ==
  In1 : Inport
  In2 : Inport  Port=2
  NAND : Subsystem
  NOT1 : Logic  Operator=NOT  IconShape=distinctive  AllPortsSameDT=off  OutDataTypeStr=boolean
  NOT2 : Logic  Operator=NOT  IconShape=distinctive  AllPortsSameDT=off  OutDataTypeStr=boolean
  Out1 : Outport
  wires:
  In1/1 -> NOT1/1
  In2/1 -> NOT2/1
  NOT1/1 -> NAND/1(In1)
  NOT2/1 -> NAND/2(In2)
  NAND/1(Out1) -> Out1/1

== system Eigth_Bit_Adder/8-BIT ADDER/ADDER5/XOR1/NAND1 ==
  In1 : Inport
  In2 : Inport  Port=2
  AND : Logic  IconShape=distinctive  AllPortsSameDT=off  OutDataTypeStr=boolean
  NOT : Logic  Operator=NOT  IconShape=distinctive  AllPortsSameDT=off  OutDataTypeStr=boolean
  Out1 : Outport
  wires:
  In2/1 -> AND/2
  NOT/1 -> Out1/1
  In1/1 -> AND/1
  AND/1 -> NOT/1

== system Eigth_Bit_Adder/8-BIT ADDER/ADDER5/XOR1/OR ==
  In1 : Inport
  In2 : Inport  Port=2
  NAND : Subsystem
  NOT1 : Logic  Operator=NOT  IconShape=distinctive  AllPortsSameDT=off  OutDataTypeStr=boolean
  NOT2 : Logic  Operator=NOT  IconShape=distinctive  AllPortsSameDT=off  OutDataTypeStr=boolean
  Out1 : Outport
  wires:
  In1/1 -> NOT1/1
  In2/1 -> NOT2/1
  NOT1/1 -> NAND/1(In1)
  NOT2/1 -> NAND/2(In2)
  NAND/1(Out1) -> Out1/1

== system Eigth_Bit_Adder/8-BIT ADDER/ADDER6/OR1/NAND ==
  In1 : Inport
  In2 : Inport  Port=2
  AND : Logic  IconShape=distinctive  AllPortsSameDT=off  OutDataTypeStr=boolean
  NOT : Logic  Operator=NOT  IconShape=distinctive  AllPortsSameDT=off  OutDataTypeStr=boolean
  Out1 : Outport
  wires:
  AND/1 -> NOT/1
  In1/1 -> AND/1
  NOT/1 -> Out1/1
  In2/1 -> AND/2

== system Eigth_Bit_Adder/8-BIT ADDER/ADDER6/XOR/NAND1 ==
  In1 : Inport
  In2 : Inport  Port=2
  AND : Logic  IconShape=distinctive  AllPortsSameDT=off  OutDataTypeStr=boolean
  NOT : Logic  Operator=NOT  IconShape=distinctive  AllPortsSameDT=off  OutDataTypeStr=boolean
  Out1 : Outport
  wires:
  In2/1 -> AND/2
  NOT/1 -> Out1/1
  In1/1 -> AND/1
  AND/1 -> NOT/1

== system Eigth_Bit_Adder/8-BIT ADDER/ADDER6/XOR/OR ==
  In1 : Inport
  In2 : Inport  Port=2
  NAND : Subsystem
  NOT1 : Logic  Operator=NOT  IconShape=distinctive  AllPortsSameDT=off  OutDataTypeStr=boolean
  NOT2 : Logic  Operator=NOT  IconShape=distinctive  AllPortsSameDT=off  OutDataTypeStr=boolean
  Out1 : Outport
  wires:
  In1/1 -> NOT1/1
  In2/1 -> NOT2/1
  NOT1/1 -> NAND/1(In1)
  NOT2/1 -> NAND/2(In2)
  NAND/1(Out1) -> Out1/1

== system Eigth_Bit_Adder/8-BIT ADDER/ADDER6/XOR1/NAND1 ==
  In1 : Inport
  In2 : Inport  Port=2
  AND : Logic  IconShape=distinctive  AllPortsSameDT=off  OutDataTypeStr=boolean
  NOT : Logic  Operator=NOT  IconShape=distinctive  AllPortsSameDT=off  OutDataTypeStr=boolean
  Out1 : Outport
  wires:
  In2/1 -> AND/2
  NOT/1 -> Out1/1
  In1/1 -> AND/1
  AND/1 -> NOT/1

== system Eigth_Bit_Adder/8-BIT ADDER/ADDER6/XOR1/OR ==
  In1 : Inport
  In2 : Inport  Port=2
  NAND : Subsystem
  NOT1 : Logic  Operator=NOT  IconShape=distinctive  AllPortsSameDT=off  OutDataTypeStr=boolean
  NOT2 : Logic  Operator=NOT  IconShape=distinctive  AllPortsSameDT=off  OutDataTypeStr=boolean
  Out1 : Outport
  wires:
  In1/1 -> NOT1/1
  In2/1 -> NOT2/1
  NOT1/1 -> NAND/1(In1)
  NOT2/1 -> NAND/2(In2)
  NAND/1(Out1) -> Out1/1

== system Eigth_Bit_Adder/8-BIT ADDER/ADDER7/OR1/NAND ==
  In1 : Inport
  In2 : Inport  Port=2
  AND : Logic  IconShape=distinctive  AllPortsSameDT=off  OutDataTypeStr=boolean
  NOT : Logic  Operator=NOT  IconShape=distinctive  AllPortsSameDT=off  OutDataTypeStr=boolean
  Out1 : Outport
  wires:
  AND/1 -> NOT/1
  In1/1 -> AND/1
  NOT/1 -> Out1/1
  In2/1 -> AND/2

== system Eigth_Bit_Adder/8-BIT ADDER/ADDER7/XOR/NAND1 ==
  In1 : Inport
  In2 : Inport  Port=2
  AND : Logic  IconShape=distinctive  AllPortsSameDT=off  OutDataTypeStr=boolean
  NOT : Logic  Operator=NOT  IconShape=distinctive  AllPortsSameDT=off  OutDataTypeStr=boolean
  Out1 : Outport
  wires:
  In2/1 -> AND/2
  NOT/1 -> Out1/1
  In1/1 -> AND/1
  AND/1 -> NOT/1

== system Eigth_Bit_Adder/8-BIT ADDER/ADDER7/XOR/OR ==
  In1 : Inport
  In2 : Inport  Port=2
  NAND : Subsystem
  NOT1 : Logic  Operator=NOT  IconShape=distinctive  AllPortsSameDT=off  OutDataTypeStr=boolean
  NOT2 : Logic  Operator=NOT  IconShape=distinctive  AllPortsSameDT=off  OutDataTypeStr=boolean
  Out1 : Outport
  wires:
  In1/1 -> NOT1/1
  In2/1 -> NOT2/1
  NOT1/1 -> NAND/1(In1)
  NOT2/1 -> NAND/2(In2)
  NAND/1(Out1) -> Out1/1

== system Eigth_Bit_Adder/8-BIT ADDER/ADDER7/XOR1/NAND1 ==
  In1 : Inport
  In2 : Inport  Port=2
  AND : Logic  IconShape=distinctive  AllPortsSameDT=off  OutDataTypeStr=boolean
  NOT : Logic  Operator=NOT  IconShape=distinctive  AllPortsSameDT=off  OutDataTypeStr=boolean
  Out1 : Outport
  wires:
  In2/1 -> AND/2
  NOT/1 -> Out1/1
  In1/1 -> AND/1
  AND/1 -> NOT/1

== system Eigth_Bit_Adder/8-BIT ADDER/ADDER7/XOR1/OR ==
  In1 : Inport
  In2 : Inport  Port=2
  NAND : Subsystem
  NOT1 : Logic  Operator=NOT  IconShape=distinctive  AllPortsSameDT=off  OutDataTypeStr=boolean
  NOT2 : Logic  Operator=NOT  IconShape=distinctive  AllPortsSameDT=off  OutDataTypeStr=boolean
  Out1 : Outport
  wires:
  In1/1 -> NOT1/1
  In2/1 -> NOT2/1
  NOT1/1 -> NAND/1(In1)
  NOT2/1 -> NAND/2(In2)
  NAND/1(Out1) -> Out1/1

== system Eigth_Bit_Adder/8-BIT ADDER/ADDER/XOR/OR/NAND ==
  In1 : Inport
  In2 : Inport  Port=2
  AND : Logic  IconShape=distinctive  AllPortsSameDT=off  OutDataTypeStr=boolean
  NOT : Logic  Operator=NOT  IconShape=distinctive  AllPortsSameDT=off  OutDataTypeStr=boolean
  Out1 : Outport
  wires:
  AND/1 -> NOT/1
  In1/1 -> AND/1
  NOT/1 -> Out1/1
  In2/1 -> AND/2

== system Eigth_Bit_Adder/8-BIT ADDER/ADDER/XOR1/OR/NAND ==
  In1 : Inport
  In2 : Inport  Port=2
  AND : Logic  IconShape=distinctive  AllPortsSameDT=off  OutDataTypeStr=boolean
  NOT : Logic  Operator=NOT  IconShape=distinctive  AllPortsSameDT=off  OutDataTypeStr=boolean
  Out1 : Outport
  wires:
  AND/1 -> NOT/1
  In1/1 -> AND/1
  NOT/1 -> Out1/1
  In2/1 -> AND/2

== system Eigth_Bit_Adder/8-BIT ADDER/ADDER1/XOR/OR/NAND ==
  In1 : Inport
  In2 : Inport  Port=2
  AND : Logic  IconShape=distinctive  AllPortsSameDT=off  OutDataTypeStr=boolean
  NOT : Logic  Operator=NOT  IconShape=distinctive  AllPortsSameDT=off  OutDataTypeStr=boolean
  Out1 : Outport
  wires:
  AND/1 -> NOT/1
  In1/1 -> AND/1
  NOT/1 -> Out1/1
  In2/1 -> AND/2

== system Eigth_Bit_Adder/8-BIT ADDER/ADDER1/XOR1/OR/NAND ==
  In1 : Inport
  In2 : Inport  Port=2
  AND : Logic  IconShape=distinctive  AllPortsSameDT=off  OutDataTypeStr=boolean
  NOT : Logic  Operator=NOT  IconShape=distinctive  AllPortsSameDT=off  OutDataTypeStr=boolean
  Out1 : Outport
  wires:
  AND/1 -> NOT/1
  In1/1 -> AND/1
  NOT/1 -> Out1/1
  In2/1 -> AND/2

== system Eigth_Bit_Adder/8-BIT ADDER/ADDER2/XOR/OR/NAND ==
  In1 : Inport
  In2 : Inport  Port=2
  AND : Logic  IconShape=distinctive  AllPortsSameDT=off  OutDataTypeStr=boolean
  NOT : Logic  Operator=NOT  IconShape=distinctive  AllPortsSameDT=off  OutDataTypeStr=boolean
  Out1 : Outport
  wires:
  AND/1 -> NOT/1
  In1/1 -> AND/1
  NOT/1 -> Out1/1
  In2/1 -> AND/2

== system Eigth_Bit_Adder/8-BIT ADDER/ADDER2/XOR1/OR/NAND ==
  In1 : Inport
  In2 : Inport  Port=2
  AND : Logic  IconShape=distinctive  AllPortsSameDT=off  OutDataTypeStr=boolean
  NOT : Logic  Operator=NOT  IconShape=distinctive  AllPortsSameDT=off  OutDataTypeStr=boolean
  Out1 : Outport
  wires:
  AND/1 -> NOT/1
  In1/1 -> AND/1
  NOT/1 -> Out1/1
  In2/1 -> AND/2

== system Eigth_Bit_Adder/8-BIT ADDER/ADDER3/XOR/OR/NAND ==
  In1 : Inport
  In2 : Inport  Port=2
  AND : Logic  IconShape=distinctive  AllPortsSameDT=off  OutDataTypeStr=boolean
  NOT : Logic  Operator=NOT  IconShape=distinctive  AllPortsSameDT=off  OutDataTypeStr=boolean
  Out1 : Outport
  wires:
  AND/1 -> NOT/1
  In1/1 -> AND/1
  NOT/1 -> Out1/1
  In2/1 -> AND/2

== system Eigth_Bit_Adder/8-BIT ADDER/ADDER3/XOR1/OR/NAND ==
  In1 : Inport
  In2 : Inport  Port=2
  AND : Logic  IconShape=distinctive  AllPortsSameDT=off  OutDataTypeStr=boolean
  NOT : Logic  Operator=NOT  IconShape=distinctive  AllPortsSameDT=off  OutDataTypeStr=boolean
  Out1 : Outport
  wires:
  AND/1 -> NOT/1
  In1/1 -> AND/1
  NOT/1 -> Out1/1
  In2/1 -> AND/2

== system Eigth_Bit_Adder/8-BIT ADDER/ADDER4/XOR/OR/NAND ==
  In1 : Inport
  In2 : Inport  Port=2
  AND : Logic  IconShape=distinctive  AllPortsSameDT=off  OutDataTypeStr=boolean
  NOT : Logic  Operator=NOT  IconShape=distinctive  AllPortsSameDT=off  OutDataTypeStr=boolean
  Out1 : Outport
  wires:
  AND/1 -> NOT/1
  In1/1 -> AND/1
  NOT/1 -> Out1/1
  In2/1 -> AND/2

== system Eigth_Bit_Adder/8-BIT ADDER/ADDER4/XOR1/OR/NAND ==
  In1 : Inport
  In2 : Inport  Port=2
  AND : Logic  IconShape=distinctive  AllPortsSameDT=off  OutDataTypeStr=boolean
  NOT : Logic  Operator=NOT  IconShape=distinctive  AllPortsSameDT=off  OutDataTypeStr=boolean
  Out1 : Outport
  wires:
  AND/1 -> NOT/1
  In1/1 -> AND/1
  NOT/1 -> Out1/1
  In2/1 -> AND/2

== system Eigth_Bit_Adder/8-BIT ADDER/ADDER5/XOR/OR/NAND ==
  In1 : Inport
  In2 : Inport  Port=2
  AND : Logic  IconShape=distinctive  AllPortsSameDT=off  OutDataTypeStr=boolean
  NOT : Logic  Operator=NOT  IconShape=distinctive  AllPortsSameDT=off  OutDataTypeStr=boolean
  Out1 : Outport
  wires:
  AND/1 -> NOT/1
  In1/1 -> AND/1
  NOT/1 -> Out1/1
  In2/1 -> AND/2

== system Eigth_Bit_Adder/8-BIT ADDER/ADDER5/XOR1/OR/NAND ==
  In1 : Inport
  In2 : Inport  Port=2
  AND : Logic  IconShape=distinctive  AllPortsSameDT=off  OutDataTypeStr=boolean
  NOT : Logic  Operator=NOT  IconShape=distinctive  AllPortsSameDT=off  OutDataTypeStr=boolean
  Out1 : Outport
  wires:
  AND/1 -> NOT/1
  In1/1 -> AND/1
  NOT/1 -> Out1/1
  In2/1 -> AND/2

== system Eigth_Bit_Adder/8-BIT ADDER/ADDER6/XOR/OR/NAND ==
  In1 : Inport
  In2 : Inport  Port=2
  AND : Logic  IconShape=distinctive  AllPortsSameDT=off  OutDataTypeStr=boolean
  NOT : Logic  Operator=NOT  IconShape=distinctive  AllPortsSameDT=off  OutDataTypeStr=boolean
  Out1 : Outport
  wires:
  AND/1 -> NOT/1
  In1/1 -> AND/1
  NOT/1 -> Out1/1
  In2/1 -> AND/2

== system Eigth_Bit_Adder/8-BIT ADDER/ADDER6/XOR1/OR/NAND ==
  In1 : Inport
  In2 : Inport  Port=2
  AND : Logic  IconShape=distinctive  AllPortsSameDT=off  OutDataTypeStr=boolean
  NOT : Logic  Operator=NOT  IconShape=distinctive  AllPortsSameDT=off  OutDataTypeStr=boolean
  Out1 : Outport
  wires:
  AND/1 -> NOT/1
  In1/1 -> AND/1
  NOT/1 -> Out1/1
  In2/1 -> AND/2

== system Eigth_Bit_Adder/8-BIT ADDER/ADDER7/XOR/OR/NAND ==
  In1 : Inport
  In2 : Inport  Port=2
  AND : Logic  IconShape=distinctive  AllPortsSameDT=off  OutDataTypeStr=boolean
  NOT : Logic  Operator=NOT  IconShape=distinctive  AllPortsSameDT=off  OutDataTypeStr=boolean
  Out1 : Outport
  wires:
  AND/1 -> NOT/1
  In1/1 -> AND/1
  NOT/1 -> Out1/1
  In2/1 -> AND/2

== system Eigth_Bit_Adder/8-BIT ADDER/ADDER7/XOR1/OR/NAND ==
  In1 : Inport
  In2 : Inport  Port=2
  AND : Logic  IconShape=distinctive  AllPortsSameDT=off  OutDataTypeStr=boolean
  NOT : Logic  Operator=NOT  IconShape=distinctive  AllPortsSameDT=off  OutDataTypeStr=boolean
  Out1 : Outport
  wires:
  AND/1 -> NOT/1
  In1/1 -> AND/1
  NOT/1 -> Out1/1
  In2/1 -> AND/2

== matlab function Eigth_Bit_Adder/MATLAB Function1 ==
  data: u input; a output; b output; c output; d output; e output; f output; g output; h output
function [a, b, c, d, e, f, g, h] = fcn(u)

    % This function breaks the elements of the list into individual inputs

    a = boolean(u(1));
    b = boolean(u(2));
    c = boolean(u(3));
    d = boolean(u(4));
    e = boolean(u(5));
    f = boolean(u(6));
    g = boolean(u(7));
    h = boolean(u(8));

end

== matlab function Eigth_Bit_Adder/MATLAB Function ==
  data: u input; a output; b output; c output; d output; e output; f output; g output; h output
function [a, b, c, d, e, f, g, h] = fcn(u)

    % This function breaks the elements of the list into individual inputs

    a = boolean(u(1));
    b = boolean(u(2));
    c = boolean(u(3));
    d = boolean(u(4));
    e = boolean(u(5));
    f = boolean(u(6));
    g = boolean(u(7));
    h = boolean(u(8));

end

== matlab function Eigth_Bit_Adder/CONVERT TO LIST ==
  data: a input; y output; b input; c input; d input; e input; f input; g input; h input
function y = fcn(a, b, c, d, e, f, g, h)

y = [a, b, c, d, e, f, g, h]

end
